simulink library "hapsrav_library"  (R2017a)
settings: Solver=VariableStepAuto  StartTime=0.0  StopTime=10.0  RelTol=1e-3
values from neighbouring files (symbols this model uses):
  absorb_h = 0:100:40000    [EnergySim.m]
  Adisk = pi * v.R_prop^2    [EnergySim.m]
  alpha_h = absorb_h    [EnergySim.m]
  aoa_data = zeros(n_cl, n)    [EnergySim.m]
  cl_bp = linspace(min_cl, max_cl,n_cl)    [EnergySim.m]
  D = [1       -.0065      288.15          0                   101325 ... (first row only)    [EnergySim.m]    (also in msn_params.m = sqrt((from_x - to_x)^2 + (from_y - to_y)^2); solar_vector.m = time.day + ut_time)
  d2r = pi / 180    (= 0.0174532925199)    [EnergySim.m]    (also in example1.m; example2.m; example3.m; example4.m)
  d_init = sqrt(dx*dx + dy*dy)    [EnergySim.m]    (also in msn_init.m)
  dchi0 = atan2(sin(dchi0), cos(dchi0))    [EnergySim.m]    (also in msn_init.m)
  dT = 0.5    [EnergySim.m]
  dT_fixed = 0.5    [EnergySim.m]
  dT_trig = 30    [EnergySim.m]
  earth_rho = 6378137.0    (= 6378137)    [EnergySim.m]
  fp = solarFP(p.orbit_rho, p.min_axis, p.orbit_dir, ic.x_ctr, ic.y_ctr, sun_az_0)    [EnergySim.m]    (also in load_fp.m = gid_tc(msn_idx).fp; solarFP.m = [1	6	2	nul eul 0	0	0	0	1	0)
  fp_coords = [x_entry y_entry]    [msn_params.m]
  fp_courses = [chi_adj nxt_chi dchi]    [msn_params.m]
  g = 9.80665    [EnergySim.m]
  Gsolar = 1367    [EnergySim.m]
  k = k+1    (= 5)    [EnergySim.m]
  K = D(:,2)    [EnergySim.m]
  lat_init = ic.lat_init_deg * obj.d2r    [EnergySim.m]
  M = time.month    [solar_vector.m]
  max_cl = max(cl_data(:))    [EnergySim.m]
  min_cl = min(cl_data(:))    [EnergySim.m]
  ND2 = load(fullfile(pwd,'nd2_data.mat'))    [EnergySim.m]    (also in nd2_data.mat = [0.0999999999999 0.200000000001 0.3 0.4 0.499999999998 0.700)
  next_init = fp(init_wp, 3)    [EnergySim.m]    (also in msn_init.m)
  pE_init = ic.pE_init    [EnergySim.m]
  pN_init = ic.pN_init    [EnergySim.m]
  r2d = 180 / pi    (= 57.2957795131)    [EnergySim.m]    (also in example1.m; example2.m; example3.m; example4.m)
  rho_SL = 1.225    [EnergySim.m]
  S = 110.4    [EnergySim.m]
  thr_lo_lim = 0.0    (= 0)    [EnergySim.m]
  time_init = struct('year', time.year, 'month', time.month,                  'day', time.day, 'hour', time.hour, 'min', time.min,                  'UTC', time.UTC)    [EnergySim.m]
  to_init = fp(init_wp, 1)    [EnergySim.m]    (also in msn_init.m)
  vgnd_init = sqrt(Vg)    [EnergySim.m]
  vtas_init = veas_init * sqrt(rho_sl/rho_alt)    [EnergySim.m]
  w_alt = 2.0 * w_alt    [EnergySim.m]
  w_xtrack = 2.0 * w_xtrack    [EnergySim.m]
undefined symbols (not defined in the file or in its folder): alpha, alpha_bp, alpha_circ, alt0_rate_init, alt_bp, alt_cmd_mode, alt_init, alt_lim_h, alt_lim_l, alt_rt_lim_periodic, cd_data, charge_eff, chi0_rate_init, chi_cmd_mode, chi_inf, chi_init, cl_data, discharge_eff, DiscIntNeverNeededParam, E_batt_max, E_init, Earth, enableFuzzyLogic, entry_init, epsln, epsln_circ, exit_init, f8_azimuth_offset, fig_eight_time, fp0, fp_coords0, fp_courses0, gamma_lim, hold_time, k_c, K_circ, lat_init_deg, lon_init_deg, max_alpha_bp, max_alt_bp, min_alpha_bp, min_alt_bp, min_axis, motor_eff, mppt_eff, num_motors, orb_dir_init, orb_len_init, orbit_dir, orbit_rho, P_acc, panel_eff, panel_vecs, phi_0, phi_lim, phi_lim_alt, phi_lim_alt_max, phi_lim_alt_min, phi_rt_lim, prop_eff_scale ... (+39)
libraries: simulink x59, hapsrav_library x9, fuzblock x3, atmospheric_library x1, aerolibtransform2 x1
(part 2 of 6)

== system hapsrav_library/Cmd - Parametric/Chi Cmd/Subsystem ==
  night_md : Inport
  chi_cmd_in : Inport  Port=2
  sun_az_rad : Inport  Port=3
  Enable : EnablePort  StatesWhenEnabling=reset
  "Azimuth angle not bounded by 0, 2pi" : Subsystem
  Circular Orbit : Subsystem  TreatAsAtomicUnit=on
  Clock : Clock
  Compare To Constant : simulink/Logic and Bit Operations/Compare To Constant  relop===  const=1  OutDataTypeStr=boolean
  Compare To Constant1 : simulink/Logic and Bit Operations/Compare To Constant  relop===  const=2  OutDataTypeStr=boolean
  Compare To Constant2 : simulink/Logic and Bit Operations/Compare To Constant  relop===  const=3  OutDataTypeStr=boolean
  Constant : Constant  Value=chi_cmd_mode
  Constant1 : Constant
  Figure Eight Orbit : Subsystem
  Merge : Merge  Inputs=3
  Racetrack Orbit : Subsystem
  Scope1 : Scope
  Switch : Switch  Criteria=u2 ~= 0
  chi_cmd : Outport
  up_or_down : Outport  Port=2
  wires:
  sun_az_rad/1 -> "Azimuth angle not bounded by 0, 2pi"/1(sun_az_rad), Figure Eight Orbit/2(sun_az_rad), Racetrack Orbit/3(sun_az_rad)
  Constant1/1 -> Switch/1
  Compare To Constant2/1 -> Figure Eight Orbit/Enable
  Constant/1 -> Switch/3
  Figure Eight Orbit/1(chi_cmd) -> Merge/3
  [t] -> Circular Orbit/2(t)
  chi_cmd_in/1 -> Circular Orbit/1(chi_cmd_in), Racetrack Orbit/2(chi_cmd_in), Figure Eight Orbit/3(chi_cmd_in)
  Switch/1 -> Compare To Constant/1, Compare To Constant1/1, Compare To Constant2/1, Scope1/1
  Circular Orbit/1(chi_cmd) -> Merge/1
  Racetrack Orbit/1(chi_cmd) -> Merge/2
  [t] -> Figure Eight Orbit/1(t)
  Compare To Constant1/1 -> Racetrack Orbit/Enable
  Compare To Constant/1 -> Circular Orbit/Enable
  [t] -> Racetrack Orbit/1(t)
  Clock/1 -> [t]
  Merge/1 -> chi_cmd/1
  night_md/1 -> Switch/2
  Racetrack Orbit/2(up_or_down) -> up_or_down/1
  "Azimuth angle not bounded by 0, 2pi"/1(2*pi*i) -> Figure Eight Orbit/4(az_offset)

== system hapsrav_library/Cmd - Parametric/Fuzzy Trajectory Optimiser Alt Cmd/Alt Rate Integrator ==
  alt_rate_cmd : Inport
  alt : Inport  Port=2
  Abs : Abs
  Compare To Constant : simulink/Logic and Bit Operations/Compare To Constant  relop=>  const=50  OutDataTypeStr=boolean
  Delay1 : Delay  DelayLength=1  InitialCondition=alt_init
  Discrete-Time Integrator : DiscreteIntegrator  IntegratorMethod=Integration: Trapezoidal  ExternalReset=rising  InitialConditionSource=external  InitialConditionSetting=State (most efficient)  SampleTime=-1  ICPrevOutput=DiscIntNeverNeededParam  ICPrevScaledInput=DiscIntNeverNeededParam
  Sum : Sum  Inputs=|+-
  alt_cmd : Outport
  wires:
  Delay1/1 -> alt_cmd/1, Discrete-Time Integrator/3, Sum/2
  Discrete-Time Integrator/1 -> Delay1/1
  alt_rate_cmd/1 -> Discrete-Time Integrator/1
  Compare To Constant/1 -> Discrete-Time Integrator/2  "trigger a reset (anti-windup)"
  alt/1 -> Sum/1
  Sum/1 -> Abs/1
  Abs/1 -> Compare To Constant/1

== system hapsrav_library/Cmd - Parametric/Fuzzy Trajectory Optimiser Chi Cmd/Subsystem ==
  chi_rate_cmd_rps : Inport
  chi : Inport  Port=2
  Abs : Abs
  Bus Creator : BusCreator  Inputs=3
  Compare To Constant : simulink/Logic and Bit Operations/Compare To Constant  relop=>  const=1000  OutDataTypeStr=boolean
  Delay1 : Delay  DelayLength=1  InitialCondition=chi_init
  Discrete-Time Integrator : DiscreteIntegrator  IntegratorMethod=Integration: Trapezoidal  ExternalReset=rising  InitialConditionSource=external  InitialConditionSetting=State (most efficient)  SampleTime=-1  ICPrevOutput=DiscIntNeverNeededParam  ICPrevScaledInput=DiscIntNeverNeededParam
  Sum : Sum  Inputs=|+-
  To Workspace1 : ToWorkspace  VariableName=pos_vector  SampleTime=-1
  chi_cmd_rad : Outport
  wires:
  Compare To Constant/1 -> Discrete-Time Integrator/2  "trigger a reset (anti-windup)"
  Sum/1 -> Abs/1
  Discrete-Time Integrator/1 -> Delay1/1
  Abs/1 -> Bus Creator/3, Compare To Constant/1
  Bus Creator/1 -> To Workspace1/1
  chi/1 -> Bus Creator/1, Sum/1
  Delay1/1 -> Discrete-Time Integrator/3, Sum/2, chi_cmd_rad/1, Bus Creator/2
  chi_rate_cmd_rps/1 -> Discrete-Time Integrator/1

== system hapsrav_library/Cmd - Parametric/Wind State/Rel Hdg ==
  wnd_dir : Inport
  psi : Inport  Port=2
  Sum : Sum  Inputs=|+-
  Trigonometric Function6 : Trigonometry
  Trigonometric Function7 : Trigonometry  Operator=cos
  Trigonometric Function8 : Trigonometry  Operator=atan2
  rel_wnd : Outport
  wires:
  Trigonometric Function6/1 -> Trigonometric Function8/1
  wnd_dir/1 -> Sum/1
  Trigonometric Function8/1 -> rel_wnd/1
  Sum/1 -> Trigonometric Function6/1, Trigonometric Function7/1
  Trigonometric Function7/1 -> Trigonometric Function8/2
  psi/1 -> Sum/2

== system hapsrav_library/Winds/Test Winds/Turn winds off at runtime ==
  Action Port : ActionPort
  East : Constant  Value=0.0
  North : Constant  Value=0.0
  Wn : Outport
  We : Outport  Port=2
  wires:
  North/1 -> Wn/1
  East/1 -> We/1

== system hapsrav_library/Winds/Test Winds/Winds ==
  day : Inport
  wmag_level : Inport  Port=2
  wdir_level : Inport  Port=3
  altitude : Inport  Port=4
  Action Port : ActionPort
  Gain : Gain  Gain=pi/180
  Product : Product
  Product1 : Product
  Trigonometric Function : Trigonometry  Operator=sincos
  Wind Direction LUT : Lookup_n-D  NumberOfTableDimensions=3  BreakpointsForDimension1=[1:1:365]  BreakpointsForDimension2=testStation.percs  BreakpointsForDimension3=testStation.alts  Table=testStation.wnd_dir  ExtrapMethod=Clip  UseLastTableValue=on  InternalRulePriority=Speed  RndMeth=Simplest  InputSameDT=on
  Wind Magnitude LUT : Lookup_n-D  NumberOfTableDimensions=3  BreakpointsForDimension1=[1:1:365]  BreakpointsForDimension2=testStation.percs  BreakpointsForDimension3=testStation.alts  Table=testStation.wnd_mag  ExtrapMethod=Clip  UseLastTableValue=on  InternalRulePriority=Speed  RndMeth=Simplest  InputSameDT=on
  Wn : Outport
  We : Outport  Port=2
  wires:
  day/1 -> Wind Direction LUT/1, Wind Magnitude LUT/1
  altitude/1 -> Wind Magnitude LUT/3, Wind Direction LUT/3
  Wind Direction LUT/1 -> Gain/1
  Gain/1 -> Trigonometric Function/1
  Trigonometric Function/2 -> [cos_dir]
  Trigonometric Function/1 -> [sin_dir]
  Wind Magnitude LUT/1 -> [w_mag]
  [w_mag] -> Product/1
  [w_mag] -> Product1/1
  [cos_dir] -> Product/2
  Product/1 -> Wn/1
  [sin_dir] -> Product1/2
  Product1/1 -> We/1
  wmag_level/1 -> Wind Magnitude LUT/2
  wdir_level/1 -> Wind Direction LUT/2

== system hapsrav_library/hapsrav_main/Kinematic 6DOF/Aero ==
  q_bar : Inport
  phi : Inport  Port=2
  gamma : Inport  Port=3
  d1Vtas : Inport  Port=4
  Vtas : Inport  Port=5
  alt : Inport  Port=6
  CL vs AoA : Subsystem
  Constant2 : Constant  Value=S
  Divide1 : Product  Inputs=**
  Thrust : Subsystem
  alpha : Outport
  theta : Outport  Port=2
  thrust : Outport  Port=3
  CL : Outport  Port=4
  CD : Outport  Port=5
  wires:
  d1Vtas/1 -> [d1Vtas]
  Divide1/1 -> [qS]
  gamma/1 -> [gamma]
  q_bar/1 -> [q_bar]
  Constant2/1 -> Divide1/2
  [q_bar] -> Divide1/1
  phi/1 -> [phi]
  Vtas/1 -> [Vtas]
  alt/1 -> [alt]
  [Vtas] -> CL vs AoA/1(Vtas)
  [gamma] -> CL vs AoA/2(gamma)
  CL vs AoA/1(CL) -> [CL]
  CL vs AoA/3(alpha) -> [alpha]
  [qS] -> CL vs AoA/3(qS)
  [alt] -> CL vs AoA/4(alt)
  CL vs AoA/4(theta) -> [theta]
  [d1Vtas] -> Thrust/1(d1Vtas)
  [phi] -> CL vs AoA/5(phi)
  [gamma] -> Thrust/2(gamma)
  [qS] -> Thrust/3(qS)
  [CL] -> Thrust/4(CL)
  Thrust/1(thrust) -> thrust/1
  [CL] -> CL/1
  [alpha] -> alpha/1
  [CD] -> Thrust/5(CD)
  [theta] -> theta/1
  CL vs AoA/2(CD) -> [CD]
  [CD] -> CD/1

== system hapsrav_library/hapsrav_main/Kinematic 6DOF/Airspeed ==
  alt : Inport
  Veas_cmd : Inport  Port=2
  s6dof0 : Inport  Port=3
  Bus Selector : BusSelector  OutputSignals=vtas0
  Constant : Constant  Value=rho_SL
  Delay1 : Delay  DelayLength=1  InitialConditionSource=Input port
      settings: InputPortMap=u0,p4
  Discrete-Time Integrator : DiscreteIntegrator  IntegratorMethod=Integration: Trapezoidal  InitialConditionSource=external  InitialConditionSetting=State (most efficient)  SampleTime=-1  ICPrevOutput=DiscIntNeverNeededParam  ICPrevScaledInput=DiscIntNeverNeededParam
  Divide2 : Product  Inputs=**
  Divide3 : Product  Inputs=**
  Divide4 : Product  Inputs=/*
  Math Function : Math  Operator=square  SaturateOnIntegerOverflow=on
  Mux1 : Mux  Inputs=2
  Saturation : Saturate  UpperLimit=1e3  LowerLimit=-1e3
  Scope : Scope
  Std Atmos : Subsystem
  Sum : Sum  Inputs=|+-
  rho_SL1 : Gain  Gain=0.5
  tau : Gain  Gain=tau_as
  vtas : Outport
  d1vtas : Outport  Port=2
  q_bar : Outport  Port=3
  Veas : Outport  Port=4
  OAT : Outport  Port=5
  wires:
  tau/1 -> Divide3/1
  [vtas0] -> Discrete-Time Integrator/2
  [veas_cmd] -> Mux1/1
  [veas_cmd] -> Sum/1
  Veas_cmd/1 -> [veas_cmd]
  [veas] -> Mux1/2
  Mux1/1 -> Scope/1
  [vtas] -> vtas/1
  [d1vtas] -> d1vtas/1
  Delay1/1 -> Divide4/2
  Divide4/1 -> [veas], Sum/2
  Discrete-Time Integrator/1 -> Delay1/1, [vtas]
  [rho_ratio] -> Divide4/1, Divide3/2
  Bus Selector/1 -> [vtas0]  "<vtas0>"
  s6dof0/1 -> Bus Selector/1
  [vtas0] -> Delay1/2
  Std Atmos/2(OAT) -> OAT/1
  [veas] -> Veas/1
  Std Atmos/1(rho_ratio) -> [rho_ratio]
  Constant/1 -> Divide2/2
  alt/1 -> Std Atmos/1(alt)
  rho_SL1/1 -> q_bar/1
  Divide2/1 -> rho_SL1/1
  Math Function/1 -> Divide2/1
  [veas] -> Math Function/1
  Sum/1 -> tau/1
  Divide3/1 -> Saturation/1
  Saturation/1 -> [d1vtas], Discrete-Time Integrator/1

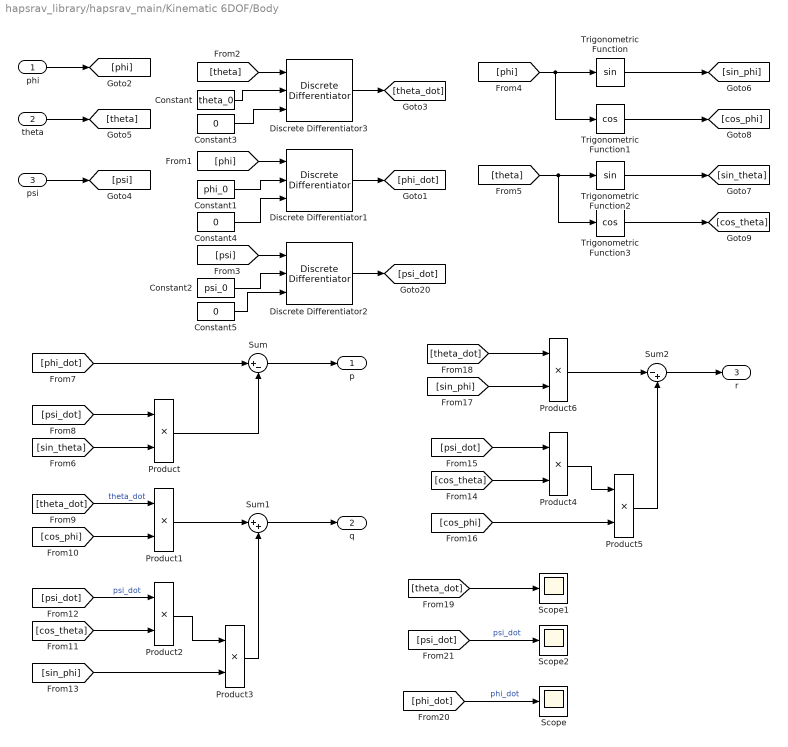
== system hapsrav_library/hapsrav_main/Kinematic 6DOF/Body ==
  phi : Inport
  theta : Inport  Port=2
  psi : Inport  Port=3
  Constant : Constant  Value=theta_0
  Constant1 : Constant  Value=phi_0
  Constant2 : Constant  Value=psi_0
  Constant3 : Constant  Value=0
  Constant4 : Constant  Value=0
  Constant5 : Constant  Value=0
  Discrete Differentiator1 : hapsrav_library/Discrete Differentiator
  Discrete Differentiator2 : hapsrav_library/Discrete Differentiator
  Discrete Differentiator3 : hapsrav_library/Discrete Differentiator
  Product{,1..6} (7 alike) : Product
  Scope : Scope
  Scope1 : Scope
  Scope2 : Scope
  Sum : Sum  Inputs=|+-
  Sum1 : Sum  Inputs=|++
  Sum2 : Sum  Inputs=|-+
  Trigonometric Function : Trigonometry
  Trigonometric Function1 : Trigonometry  Operator=cos
  Trigonometric Function2 : Trigonometry
  Trigonometric Function3 : Trigonometry  Operator=cos
  p : Outport
  q : Outport  Port=2
  r : Outport  Port=3
  wires:
  [theta_dot] -> Scope1/1
  Constant5/1 -> Discrete Differentiator2/3
  Constant4/1 -> Discrete Differentiator1/3
  Constant3/1 -> Discrete Differentiator3/3
  [psi_dot] -> Scope2/1  "psi_dot"
  [phi_dot] -> Scope/1  "phi_dot"
  Constant/1 -> Discrete Differentiator3/2
  psi/1 -> [psi]
  theta/1 -> [theta]
  phi/1 -> [phi]
  [phi] -> Trigonometric Function1/1, Trigonometric Function/1
  [theta] -> Trigonometric Function3/1, Trigonometric Function2/1
  Trigonometric Function3/1 -> [cos_theta]
  Trigonometric Function2/1 -> [sin_theta]
  Trigonometric Function1/1 -> [cos_phi]
  Trigonometric Function/1 -> [sin_phi]
  [sin_theta] -> Product/2
  [psi_dot] -> Product/1
  [phi_dot] -> Sum/1
  Product/1 -> Sum/2
  Sum/1 -> p/1
  [theta_dot] -> Product1/1  "theta_dot"
  [cos_phi] -> Product1/2
  [cos_theta] -> Product2/2
  [psi_dot] -> Product2/1  "psi_dot"
  Product2/1 -> Product3/1
  [sin_phi] -> Product3/2
  Product1/1 -> Sum1/1
  Product3/1 -> Sum1/2
  Sum1/1 -> q/1
  [cos_theta] -> Product4/2
  [psi_dot] -> Product4/1
  Product4/1 -> Product5/1
  [cos_phi] -> Product5/2
  Product5/1 -> Sum2/2
  [theta_dot] -> Product6/1
  [sin_phi] -> Product6/2
  Product6/1 -> Sum2/1
  Sum2/1 -> r/1
  Discrete Differentiator3/1 -> [theta_dot]
  [theta] -> Discrete Differentiator3/1
  [phi] -> Discrete Differentiator1/1
  Constant1/1 -> Discrete Differentiator1/2
  Discrete Differentiator1/1 -> [phi_dot]
  Constant2/1 -> Discrete Differentiator2/2
  [psi] -> Discrete Differentiator2/1
  Discrete Differentiator2/1 -> [psi_dot]

== system hapsrav_library/hapsrav_main/Kinematic 6DOF/EAS Cmd Filter ==
  eas cmd : Inport
  s6dof0 : Inport  Port=2
  1/tau : Gain  Gain=0.1
  Bus Selector : BusSelector  OutputSignals=veas0
  Delay1 : Delay  DelayLength=1  InitialConditionSource=Input port
      settings: InputPortMap=u0,p4
  Discrete-Time Integrator : DiscreteIntegrator  IntegratorMethod=Integration: Trapezoidal  InitialConditionSource=external  InitialConditionSetting=State (most efficient)  SampleTime=-1  ICPrevOutput=DiscIntNeverNeededParam  ICPrevScaledInput=DiscIntNeverNeededParam
  Saturation : Saturate  UpperLimit=veas_rt_lim  LowerLimit=-veas_rt_lim
  Sum : Sum  Inputs=|+-
  filt eas cmd : Outport
  wires:
  Saturation/1 -> Discrete-Time Integrator/1
  1/tau/1 -> Saturation/1
  Sum/1 -> 1/tau/1
  Discrete-Time Integrator/1 -> filt eas cmd/1, Delay1/1
  eas cmd/1 -> Sum/1
  Delay1/1 -> Sum/2
  [eas_init] -> Discrete-Time Integrator/2
  [eas_init] -> Delay1/2
  Bus Selector/1 -> [eas_init]  "<veas0>"
  s6dof0/1 -> Bus Selector/1

== system hapsrav_library/hapsrav_main/Kinematic 6DOF/Idle Pwr ==
  thrust : Inport
  hdot : Inport  Port=2
  vdot : Inport  Port=3
  Constant1 : Constant  Value=THRUST_REVERSAL
  Constant2 : Constant  Value=thrust0
  Data Type Conversion : DataTypeConversion  OutDataTypeStr=double
  Data Type Conversion1 : DataTypeConversion  OutDataTypeStr=double
  Decel Detection : Stateflow chart  TreatAsAtomicUnit=on
  Delay1 : Delay  DelayLength=1  InitialConditionSource=Input port
      settings: InputPortMap=u0,p4
  Descent Detection : Stateflow chart  TreatAsAtomicUnit=on
  Logical Operator : Logic  Operator=NOT  AllPortsSameDT=off  OutDataTypeStr=boolean
  Logical Operator1 : Logic  AllPortsSameDT=off  OutDataTypeStr=boolean
  Logical Operator2 : Logic  AllPortsSameDT=off  OutDataTypeStr=boolean
  Scope : Scope
  Scope1 : Scope  NumInputPorts=2
  Terminator : Terminator
  Terminator1 : Terminator
  idleDesc : Outport
  wires:
  Data Type Conversion1/1 -> idleDesc/1
  Data Type Conversion/1 -> Terminator1/1
  Logical Operator1/1 -> Data Type Conversion/1
  [idle_descent] -> Logical Operator2/2
  Logical Operator2/1 -> Data Type Conversion1/1
  [idle_decel] -> Logical Operator1/1
  Logical Operator/1 -> Logical Operator2/1, Logical Operator1/2
  [idle_decel] -> Scope1/1
  Descent Detection/2(idleDesc) -> [idle_descent]
  Constant1/1 -> Logical Operator/1
  [thrust] -> Scope1/2
  Decel Detection/1(spd_flag) -> Scope/1
  Decel Detection/2(idleDecel) -> [idle_decel]
  [thrust] -> Decel Detection/2(thrust)
  [vdot] -> Decel Detection/1(vdot)
  Descent Detection/1(alt_flag) -> Terminator/1
  [hdot] -> Descent Detection/1(hdot)
  [thrust] -> Descent Detection/2(thrust)
  Delay1/1 -> [thrust]
  Constant2/1 -> Delay1/2
  thrust/1 -> Delay1/1
  hdot/1 -> [hdot]
  vdot/1 -> [vdot]

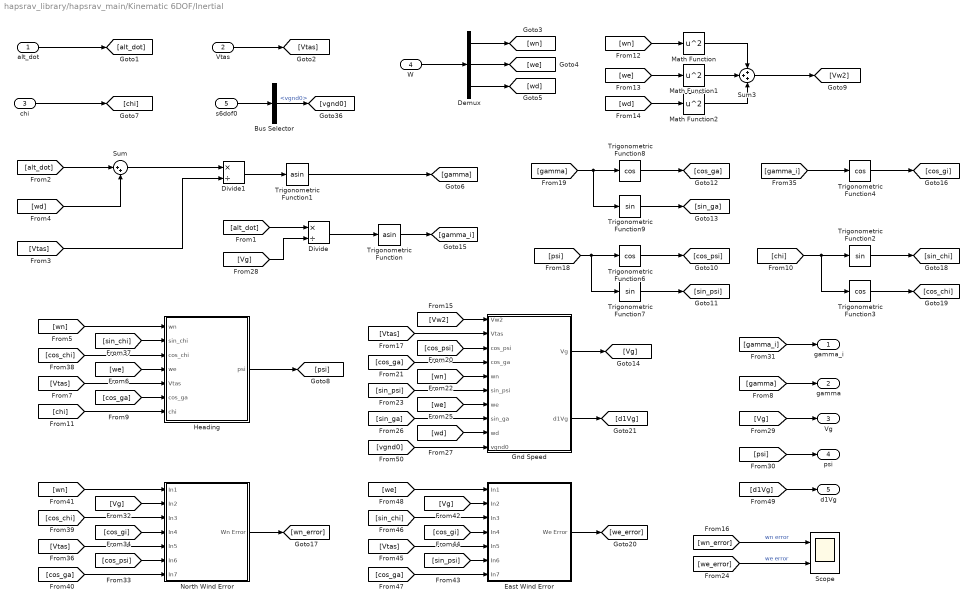
== system hapsrav_library/hapsrav_main/Kinematic 6DOF/Inertial ==
  alt_dot : Inport
  Vtas : Inport  Port=2
  chi : Inport  Port=3
  W : Inport  Port=4
  s6dof0 : Inport  Port=5
  Bus Selector : BusSelector  OutputSignals=vgnd0
  Demux : Demux  Outputs=3
  Divide : Product  Inputs=*/
  Divide1 : Product  Inputs=*/
  East Wind Error : Subsystem
  Gnd Speed : Subsystem
  Heading : Subsystem
  Math Function : Math  Operator=square  SaturateOnIntegerOverflow=on
  Math Function1 : Math  Operator=square  SaturateOnIntegerOverflow=on
  Math Function2 : Math  Operator=square  SaturateOnIntegerOverflow=on
  North Wind Error : Subsystem
  Scope : Scope  NumInputPorts=2
  Sum : Sum  Inputs=|++
  Sum3 : Sum  Inputs=+++
  Trigonometric Function : Trigonometry  Operator=asin
  Trigonometric Function1 : Trigonometry  Operator=asin
  Trigonometric Function2 : Trigonometry
  Trigonometric Function{3..4,6,8} (4 alike) : Trigonometry  Operator=cos
  Trigonometric Function7 : Trigonometry
  Trigonometric Function9 : Trigonometry
  gamma_i : Outport
  gamma : Outport  Port=2
  Vg : Outport  Port=3
  psi : Outport  Port=4
  d1Vg : Outport  Port=5
  wires:
  [Vg] -> Divide/2
  Divide/1 -> Trigonometric Function/1
  alt_dot/1 -> [alt_dot]
  [alt_dot] -> Divide/1
  [alt_dot] -> Sum/1
  [wd] -> Sum/2
  Sum/1 -> Divide1/1
  Vtas/1 -> [Vtas]
  [Vtas] -> Divide1/2
  Divide1/1 -> Trigonometric Function1/1
  Trigonometric Function1/1 -> [gamma]
  W/1 -> Demux/1
  Demux/1 -> [wn]
  Demux/2 -> [we]
  Demux/3 -> [wd]
  [gamma] -> gamma/1
  chi/1 -> [chi]
  [chi] -> Trigonometric Function3/1, Trigonometric Function2/1
  [wn] -> Math Function/1
  [we] -> Math Function1/1
  [wd] -> Math Function2/1
  Math Function/1 -> Sum3/1
  Math Function1/1 -> Sum3/2
  Math Function2/1 -> Sum3/3
  Sum3/1 -> [Vw2]
  [psi] -> Trigonometric Function7/1, Trigonometric Function6/1
  Trigonometric Function6/1 -> [cos_psi]
  Trigonometric Function7/1 -> [sin_psi]
  Trigonometric Function8/1 -> [cos_ga]
  Trigonometric Function9/1 -> [sin_ga]
  [gamma] -> Trigonometric Function9/1, Trigonometric Function8/1
  [Vg] -> Vg/1
  [psi] -> psi/1
  Trigonometric Function/1 -> [gamma_i]
  [gamma_i] -> gamma_i/1
  Trigonometric Function4/1 -> [cos_gi]
  [gamma_i] -> Trigonometric Function4/1
  Trigonometric Function2/1 -> [sin_chi]
  Trigonometric Function3/1 -> [cos_chi]
  [wn] -> Heading/1(wn)
  [sin_chi] -> Heading/2(sin_chi)
  [cos_chi] -> Heading/3(cos_chi)
  [we] -> Heading/4(we)
  [Vtas] -> Heading/5(Vtas)
  [cos_ga] -> Heading/6(cos_ga)
  [chi] -> Heading/7(chi)
  Heading/1(psi) -> [psi]
  [Vw2] -> Gnd Speed/1(Vw2)
  [Vtas] -> Gnd Speed/2(Vtas)
  [cos_psi] -> Gnd Speed/3(cos_psi)
  [cos_ga] -> Gnd Speed/4(cos_ga)
  [wn] -> Gnd Speed/5(wn)
  [sin_psi] -> Gnd Speed/6(sin_psi)
  [we] -> Gnd Speed/7(we)
  [sin_ga] -> Gnd Speed/8(sin_ga)
  [wd] -> Gnd Speed/9(wd)
  Gnd Speed/1(Vg) -> [Vg]
  [wn] -> North Wind Error/1(In1)
  [Vg] -> North Wind Error/2(In2)
  [cos_chi] -> North Wind Error/3(In3)
  [cos_gi] -> North Wind Error/4(In4)
  [Vtas] -> North Wind Error/5(In5)
  [cos_psi] -> North Wind Error/6(In6)
  [cos_ga] -> North Wind Error/7(In7)
  [sin_psi] -> East Wind Error/6(In6)
  [cos_ga] -> East Wind Error/7(In7)
  [Vtas] -> East Wind Error/5(In5)
  [cos_gi] -> East Wind Error/4(In4)
  [sin_chi] -> East Wind Error/3(In3)
  [Vg] -> East Wind Error/2(In2)
  [we] -> East Wind Error/1(In1)
  North Wind Error/1(Wn Error) -> [wn_error]
  East Wind Error/1(We Error) -> [we_error]
  [wn_error] -> Scope/1  "wn error"
  [we_error] -> Scope/2  "we error"
  Gnd Speed/2(d1Vg) -> [d1Vg]
  [d1Vg] -> d1Vg/1
  [vgnd0] -> Gnd Speed/10(vgnd0)
  Bus Selector/1 -> [vgnd0]  "<vgnd0>"
  s6dof0/1 -> Bus Selector/1

== system hapsrav_library/hapsrav_main/Kinematic 6DOF/Initial Conditions ==
  Bus Creator : BusCreator  Inputs='alt0','veas0','phi0','theta0','chi0','vgnd0','altRt0','vtas0'
  Constant : Constant  Value=pE_init
  Constant1 : Constant  Value=alt_init
  Constant10 : Constant  Value=theta_0
  Constant2 : Constant  Value=veas_init
  Constant3 : Constant  Value=chi_init
  Constant4 : Constant  Value=vgnd_init
  Constant5 : Constant  Value=vtas_init
  Constant7 : Constant  Value=alt0_rate_init
  Constant8 : Constant  Value=pN_init
  Constant9 : Constant  Value=phi_0
  Mux : Mux  Inputs=2
  s6dof0 : Outport
  posn0 : Outport  Port=2
  wires:
  Constant5/1 -> Bus Creator/8  "vtas0"
  Constant8/1 -> Mux/2  "pN_0"
  Constant/1 -> Mux/1  "pE_0"
  Bus Creator/1 -> s6dof0/1
  Constant1/1 -> Bus Creator/1  "alt0"
  Constant2/1 -> Bus Creator/2  "veas0"
  Constant9/1 -> Bus Creator/3  "phi0"
  Constant10/1 -> Bus Creator/4  "theta0"
  Constant3/1 -> Bus Creator/5  "chi0"
  Constant4/1 -> Bus Creator/6  "vgnd0"
  Constant7/1 -> Bus Creator/7  "altRt0"
  Mux/1 -> posn0/1

== system hapsrav_library/hapsrav_main/Kinematic 6DOF/Navigation ==
  Va : Inport
  psi : Inport  Port=2
  W : Inport  Port=3
  alt : Inport  Port=4
  posn0 : Inport  Port=5
  Demux : Demux  Outputs=3
  Demux1 : Demux  Outputs=2
  Flat Earth to LLA : Subsystem  Commented=on
  Flat Earth to LLA Aero BLockset : Subsystem
  NED Posn : Subsystem
  Terminator : Terminator
  Terminator3 : Terminator
  Terminator4 : Terminator
  pN : Outport
  pE : Outport  Port=2
  lat_deg : Outport  Port=3
  lon_deg : Outport  Port=4
  wires:
  Va/1 -> [Va]
  psi/1 -> [psi]
  W/1 -> Demux/1
  Demux/1 -> [wn]
  Demux/2 -> [we]
  Demux/3 -> Terminator/1
  [Va] -> NED Posn/1(Va)
  [psi] -> NED Posn/2(psi)
  [we] -> NED Posn/3(we)
  [wn] -> NED Posn/4(wn)
  NED Posn/2(pE_dot) -> Terminator3/1
  NED Posn/4(pN_dot) -> Terminator4/1
  alt/1 -> [alt]
  Demux1/1 -> NED Posn/5(pE0)
  Demux1/2 -> NED Posn/6(pN0)
  NED Posn/1(pE) -> [pE]
  NED Posn/3(pN) -> [pN]
  [pE] -> pE/1
  [pN] -> pN/1
  Flat Earth to LLA Aero BLockset/1(lat_deg) -> lat_deg/1
  [alt] -> Flat Earth to LLA Aero BLockset/1(alt)
  [pN] -> Flat Earth to LLA Aero BLockset/2(pN)
  [pE] -> Flat Earth to LLA Aero BLockset/3(pE)
  Flat Earth to LLA Aero BLockset/2(lon_deg) -> lon_deg/1
  posn0/1 -> Demux1/1

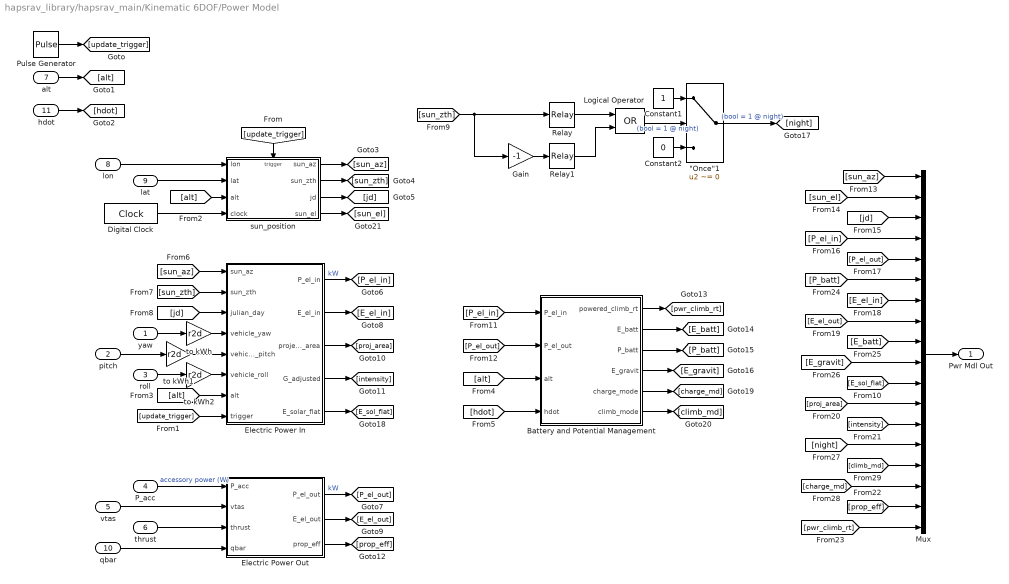
== system hapsrav_library/hapsrav_main/Kinematic 6DOF/Power Model ==
  yaw : Inport
  pitch : Inport  Port=2
  roll : Inport  Port=3
  P_acc : Inport  Port=4
  vtas : Inport  Port=5
  thrust : Inport  Port=6
  alt : Inport  Port=7
  lon : Inport  Port=8
  lat : Inport  Port=9
  qbar : Inport  Port=10
  hdot : Inport  Port=11
  "\"Once\"1" : Switch  Criteria=u2 ~= 0
  Battery and Potential Management : Subsystem
  Constant1 : Constant
  Constant2 : Constant  Value=0
  Digital Clock : DigitalClock  SampleTime=dT_fixed
  Electric Power In : Subsystem
  Electric Power Out : Subsystem
  Gain : Gain  Gain=-1
  Logical Operator : Logic  Operator=OR  AllPortsSameDT=off  OutDataTypeStr=boolean
  Mux : Mux  Inputs=18
  Pulse Generator : DiscretePulseGenerator  Period=dT_trig*2/dT_fixed  PulseWidth=dT_trig/dT_fixed  PhaseDelay=1  SampleTime=dT_fixed
  Relay : Relay  OnSwitchValue=90  OffSwitchValue=89.5
  Relay1 : Relay  OnSwitchValue=90  OffSwitchValue=89.5
  sun_position : Subsystem  TreatAsAtomicUnit=on
  to kWh : Gain  Gain=r2d
  to kWh1 : Gain  Gain=r2d
  to kWh2 : Gain  Gain=r2d
  Pwr Mdl Out : Outport
  wires:
  roll/1 -> to kWh2/1
  yaw/1 -> to kWh/1
  P_acc/1 -> Electric Power Out/1(P_acc)  "accessory power (W)"
  Battery and Potential Management/1(powered_climb_rt) -> [pwr_climb_rt]
  vtas/1 -> Electric Power Out/2(vtas)
  pitch/1 -> to kWh1/1
  lon/1 -> sun_position/1(lon)
  lat/1 -> sun_position/2(lat)
  to kWh/1 -> Electric Power In/4(vehicle_yaw)
  to kWh1/1 -> Electric Power In/5(vehicle_pitch)
  to kWh2/1 -> Electric Power In/6(vehicle_roll)
  qbar/1 -> Electric Power Out/4(qbar)
  Digital Clock/1 -> sun_position/4(clock)
  Pulse Generator/1 -> [update_trigger]
  [update_trigger] -> sun_position/Trigger
  [update_trigger] -> Electric Power In/8(trigger)
  alt/1 -> [alt]
  [alt] -> sun_position/3(alt)
  [alt] -> Electric Power In/7(alt)
  [alt] -> Battery and Potential Management/3(alt)
  "\"Once\"1"/1 -> [night]  "(bool = 1 @ night)"
  Relay1/1 -> Logical Operator/2
  Relay/1 -> Logical Operator/1
  Gain/1 -> Relay1/1
  Constant1/1 -> "\"Once\"1"/1
  Constant2/1 -> "\"Once\"1"/3
  Logical Operator/1 -> "\"Once\"1"/2  "(bool = 1 @ night)"
  hdot/1 -> [hdot]
  [hdot] -> Battery and Potential Management/4(hdot)
  thrust/1 -> Electric Power Out/3(thrust)
  sun_position/1(sun_az) -> [sun_az]
  sun_position/3(jd) -> [jd]
  sun_position/2(sun_zth) -> [sun_zth]
  [sun_az] -> Electric Power In/1(sun_az)
  [sun_zth] -> Electric Power In/2(sun_zth)
  [jd] -> Electric Power In/3(julian_day)
  [sun_zth] -> Gain/1, Relay/1
  Electric Power In/1(P_el_in) -> [P_el_in]  "kW"
  Electric Power Out/1(P_el_out) -> [P_el_out]  "kW"
  [P_el_in] -> Battery and Potential Management/1(P_el_in)
  [P_el_out] -> Battery and Potential Management/2(P_el_out)
  Electric Power In/2(E_el_in) -> [E_el_in]
  Electric Power Out/2(E_el_out) -> [E_el_out]
  Electric Power In/3(projected_area) -> [proj_area]
  Electric Power In/4(G_adjusted) -> [intensity]
  Electric Power Out/3(prop_eff) -> [prop_eff]
  Battery and Potential Management/2(E_batt) -> [E_batt]
  Battery and Potential Management/3(P_batt) -> [P_batt]
  Battery and Potential Management/4(E_gravit) -> [E_gravit]
  Mux/1 -> Pwr Mdl Out/1
  Electric Power In/5(E_solar_flat) -> [E_sol_flat]
  Battery and Potential Management/6(climb_mode) -> [climb_md]
  Battery and Potential Management/5(charge_mode) -> [charge_md]
  sun_position/4(sun_el) -> [sun_el]
  [sun_az] -> Mux/1
  [sun_el] -> Mux/2
  [jd] -> Mux/3
  [P_el_in] -> Mux/4
  [P_el_out] -> Mux/5
  [P_batt] -> Mux/6
  [E_el_in] -> Mux/7
  [E_el_out] -> Mux/8
  [E_batt] -> Mux/9
  [E_gravit] -> Mux/10
  [E_sol_flat] -> Mux/11
  [proj_area] -> Mux/12
  [intensity] -> Mux/13
  [night] -> Mux/14
  [climb_md] -> Mux/15
  [charge_md] -> Mux/16
  [prop_eff] -> Mux/17
  [pwr_climb_rt] -> Mux/18

== system hapsrav_library/hapsrav_main/Kinematic 6DOF/Selectable Modes ==
  mode : Inport
  vl_cmds : Inport  Port=2
  Vg : Inport  Port=3
  d1Vg : Inport  Port=4
  s6dof0 : Inport  Port=5
  idleDesc : Inport  Port=6
  Constant2 : Constant  Value=gamma_lim
  Divide : Product  Inputs=**
  Gain : Gain  Gain=-1
  Logical Operator : Logic  Operator=NOT  AllPortsSameDT=off  OutDataTypeStr=boolean
  Merge : Merge  InitialOutput=alt_init
  Merge1 : Merge  InitialOutput=alt0_rate_init
  Merge2 : Merge  InitialOutput=phi_0
  Merge3 : Merge  InitialOutput=chi_init
  Trajectory_Optimization : Subsystem  TreatAsAtomicUnit=on
  Trigonometric Function : Trigonometry
  Waypoint_Navigation : Subsystem  TreatAsAtomicUnit=on
  alt : Outport
  d1alt : Outport  Port=2
  phi : Outport  Port=3
  chi : Outport  Port=4
  wires:
  [idleDesc] -> Waypoint_Navigation/7(idleDesc)
  [max_desc_rt] -> Waypoint_Navigation/6(max_desc_rt)
  [max_desc_rt] -> Trajectory_Optimization/5(max_desc_rt)
  [Vg] -> Divide/2
  Trigonometric Function/1 -> Divide/1
  Divide/1 -> [max_desc_rt], Gain/1
  Constant2/1 -> Trigonometric Function/1
  idleDesc/1 -> [idleDesc]
  [idleDesc] -> Trajectory_Optimization/6(idleDesc)
  mode/1 -> Logical Operator/1, Waypoint_Navigation/Enable
  Logical Operator/1 -> Trajectory_Optimization/Enable
  Trajectory_Optimization/4(chi) -> [b_chi]
  Trajectory_Optimization/1(alt) -> [b_alt]
  Trajectory_Optimization/2(d1alt) -> [b_d1alt]
  Trajectory_Optimization/3(phi) -> [b_phi]
  Waypoint_Navigation/1(alt) -> [a_alt]
  Waypoint_Navigation/2(d1alt) -> [a_d1alt]
  Waypoint_Navigation/3(phi) -> [a_phi]
  Waypoint_Navigation/4(chi) -> [a_chi]
  Merge/1 -> alt/1
  Merge1/1 -> d1alt/1
  Merge2/1 -> phi/1
  Merge3/1 -> chi/1
  [a_alt] -> Merge/1
  [b_alt] -> Merge/2
  [b_d1alt] -> Merge1/2
  [a_d1alt] -> Merge1/1
  [a_phi] -> Merge2/1
  [b_phi] -> Merge2/2
  [b_chi] -> Merge3/2
  [a_chi] -> Merge3/1
  vl_cmds/1 -> [vl_cmds]
  Vg/1 -> [Vg]
  d1Vg/1 -> [d1Vg]
  [vl_cmds] -> Waypoint_Navigation/1(vert_lat_cmds)
  [Vg] -> Waypoint_Navigation/2(Vg)
  [d1Vg] -> Waypoint_Navigation/3(d1Vg)
  [max_clmb_rt] -> Trajectory_Optimization/4(max_clmb_rt)
  [Vg] -> Trajectory_Optimization/2(Vg)
  [vl_cmds] -> Trajectory_Optimization/1(vert_lat_cmds)
  s6dof0/1 -> [ICs]
  [ICs] -> Trajectory_Optimization/3(s6dof0)
  [ICs] -> Waypoint_Navigation/4(s6dof0)
  [max_clmb_rt] -> Waypoint_Navigation/5(max_clmb_rt)
  Gain/1 -> [max_clmb_rt]

== system hapsrav_library/hapsrav_main/Outputs/Negative Gnd Speed ==
  psi : Inport
  gamma : Inport  Port=2
  Vtas : Inport  Port=3
  Vg : Inport  Port=4
  Abs : Abs
  Compare To Constant : simulink/Logic and Bit Operations/Compare To Constant  relop=>  const=pi/2  OutDataTypeStr=boolean
  Compare To Constant1 : simulink/Logic and Bit Operations/Compare To Constant  relop=<=  const=Wmag  OutDataTypeStr=boolean
  Constant : Constant  Value=-1
  Constant1 : Constant  Value=Wmag
  Constant2 : Constant  Value=Wn
  Constant3 : Constant
  Constant4 : Constant  Value=We
  Constant5 : Constant  Value=Wd
  Divide : Product  Inputs=*/
  Divide1 : Product  Inputs=**
  Dot Product : DotProduct  InputSameDT=on  OutDataTypeStr=Inherit: Inherit via internal rule
  Gain : Gain  Gain=-1
  Logical Operator1 : Logic  AllPortsSameDT=off  OutDataTypeStr=boolean
  Mux : Mux  Inputs=3
  Mux1 : Mux  Inputs=3
  Product{,1..3} (4 alike) : Product
  Reshape : Reshape  OutputDimensionality=Row vector (2-D)
  Scope : Scope
  Switch : Switch  Criteria=u2 > Threshold
  Trigonometric Function : Trigonometry  Operator=sincos
  Trigonometric Function4 : Trigonometry  Operator=acos
  Trigonometric Function5 : Trigonometry  Operator=sincos
  Vg_out : Outport
  wires:
  psi/1 -> Trigonometric Function/1
  gamma/1 -> Trigonometric Function5/1
  Trigonometric Function5/1 -> Gain/1
  Gain/1 -> Mux/3
  Mux/1 -> Product2/2
  Product2/1 -> Dot Product/1
  Dot Product/1 -> Divide/1
  Vtas/1 -> [Vtas]
  [Vtas] -> Product2/1
  [Vtas] -> Divide1/1
  Divide1/1 -> Divide/2
  Constant1/1 -> Divide1/2
  Divide/1 -> Trigonometric Function4/1
  Trigonometric Function5/2 -> Product/2, Product1/1
  Trigonometric Function4/1 -> Abs/1
  Abs/1 -> Compare To Constant/1
  [Vtas] -> Compare To Constant1/1
  Compare To Constant1/1 -> Scope/1, Logical Operator1/2
  Compare To Constant/1 -> Logical Operator1/1
  Logical Operator1/1 -> Switch/2
  Constant/1 -> Switch/1
  Constant3/1 -> Switch/3
  Switch/1 -> Product3/2
  Vg/1 -> Product3/1
  Product3/1 -> Vg_out/1
  Trigonometric Function/2 -> Product/1
  Trigonometric Function/1 -> Product1/2
  Product1/1 -> Mux/2
  Product/1 -> Mux/1
  Mux1/1 -> Reshape/1
  Constant2/1 -> Mux1/1
  Constant4/1 -> Mux1/2
  Constant5/1 -> Mux1/3
  Reshape/1 -> Dot Product/2

== system hapsrav_library/Cmd - Parametric/Chi Cmd/Flight Plan/D2N ==
  leg_state : Inport
  av_state : Inport  Port=2
  Bus Selector : BusSelector  OutputSignals=av_posn
  Bus Selector1 : BusSelector  OutputSignals=leg_coords.to_x,leg_coords.to_y
  Demux1 : Demux
  Display1 : Display
  Distance : Subsystem  TreatAsAtomicUnit=on
  Memory5 : Memory  X0=d_init
  Terminator2 : Terminator
  Terminator3 : Terminator
  av_d2n : Outport
  wires:
  [to_y] -> Distance/3(to_y)
  [av_y] -> Distance/4(from_y)
  [av_x] -> Distance/2(from_x)
  [to_x] -> Distance/1(to_x)
  Bus Selector1/1 -> [to_x]  "<to_x>"
  Bus Selector1/2 -> [to_y]  "<to_y>"
  leg_state/1 -> Bus Selector1/1
  Memory5/1 -> av_d2n/1
  Demux1/4 -> Terminator3/1
  Demux1/3 -> Terminator2/1
  [av_d2n] -> Memory5/1
  Bus Selector/1 -> Demux1/1  "<av_posn>"
  av_state/1 -> Bus Selector/1
  Demux1/1 -> [av_x]
  Demux1/2 -> [av_y]
  Distance/1(Dist) -> Display1/1, [av_d2n]

== system hapsrav_library/Cmd - Parametric/Chi Cmd/Flight Plan/Mission Command ==
  orbit_state : Inport
  leg_state : Inport  Port=2
  av_state : Inport  Port=3
  nav_mode : Inport  Port=4
  Compare To Zero : simulink/Logic and Bit Operations/Compare To Zero  relop===  OutDataTypeStr=boolean
  Compare To Zero1 : simulink/Logic and Bit Operations/Compare To Zero  relop=>  OutDataTypeStr=boolean
  Entry Mode : Subsystem
  Merge{,1..3} (4 alike) : Merge
  Not Entry Mode : Subsystem
  Terminator : Terminator
  chi_cmd : Outport
  chi_d : Outport  Port=2
  sweep : Outport  Port=3
  wires:
  [sweep_1] -> Merge3/2
  [sweep_0] -> Merge3/1
  Merge3/1 -> sweep/1
  Not Entry Mode/4(sweep) -> [sweep_1]
  Entry Mode/4(sweep) -> [sweep_0]
  [orbit_state] -> Not Entry Mode/1(orbit_state)
  orbit_state/1 -> [orbit_state]
  [nav_mode] -> Not Entry Mode/4(nav_mode)
  [av_state] -> Not Entry Mode/3(av_state)
  [xtrack_1] -> Merge2/2
  [xtrack_0] -> Merge2/1
  [chi_d_1] -> Merge1/2
  [chi_cmd_1] -> Merge/2
  Not Entry Mode/3(xtrack) -> [xtrack_1]
  Not Entry Mode/2(chi_d) -> [chi_d_1]
  Not Entry Mode/1(chi_cmd) -> [chi_cmd_1]
  [chi_d_0] -> Merge1/1
  [chi_cmd_0] -> Merge/1
  Entry Mode/3(xtrack) -> [xtrack_0]
  Entry Mode/2(chi_d) -> [chi_d_0]
  Entry Mode/1(chi_cmd) -> [chi_cmd_0]
  Merge2/1 -> Terminator/1
  Merge1/1 -> chi_d/1
  Merge/1 -> chi_cmd/1
  [av_state] -> Entry Mode/2(av_state)
  [leg_state] -> Entry Mode/1(leg_state)
  Compare To Zero/1 -> Entry Mode/Enable
  [nav_mode] -> Compare To Zero1/1
  [nav_mode] -> Compare To Zero/1
  Compare To Zero1/1 -> Not Entry Mode/Enable
  nav_mode/1 -> [nav_mode]
  [leg_state] -> Not Entry Mode/2(leg_state)
  leg_state/1 -> [leg_state]
  av_state/1 -> [av_state]

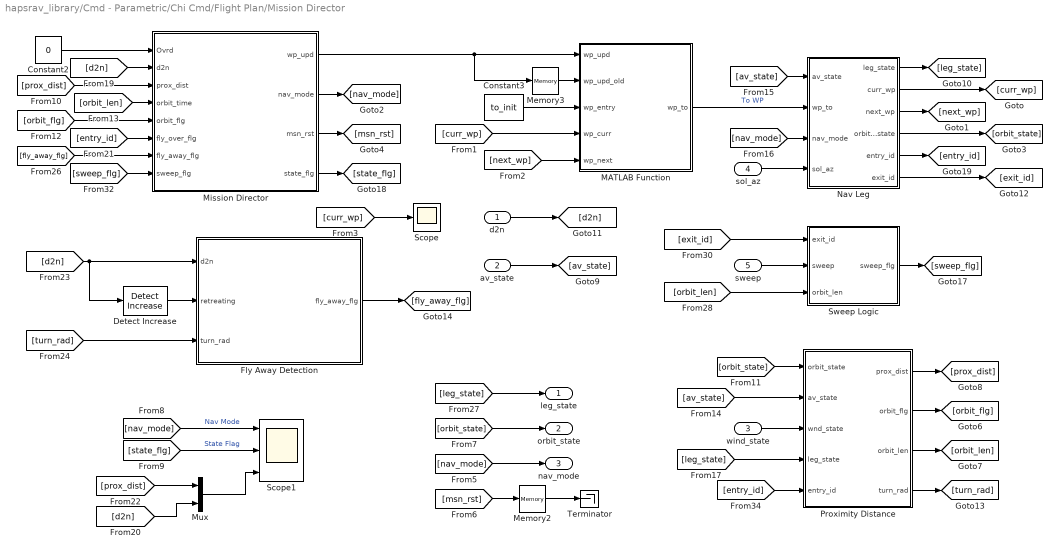
== system hapsrav_library/Cmd - Parametric/Chi Cmd/Flight Plan/Mission Director ==
  d2n : Inport
  av_state : Inport  Port=2
  wind_state : Inport  Port=3
  sol_az : Inport  Port=4
  sweep : Inport  Port=5
  Constant2 : Constant  Value=0
  Constant3 : Constant  Value=to_init
  Detect Increase : simulink/Logic and Bit Operations/Detect Increase  vinit=0.0  OutDataTypeStr=boolean
  Fly Away Detection : Stateflow chart  TreatAsAtomicUnit=on
  MATLAB Function : MATLAB Function  TreatAsAtomicUnit=on
  Memory2 : Memory  X0=1
  Memory3 : Memory  X0=-1
  Mission Director : Stateflow chart  TreatAsAtomicUnit=on
  Mux : Mux  Inputs=2
  Nav Leg : Subsystem
  Proximity Distance : Subsystem
  Scope : Scope
  Scope1 : Scope  NumInputPorts=3
  Sweep Logic : Subsystem
  Terminator : Terminator
  leg_state : Outport
  orbit_state : Outport  Port=2
  nav_mode : Outport  Port=3
  wires:
  Memory2/1 -> Terminator/1
  sol_az/1 -> Nav Leg/4(sol_az)
  [curr_wp] -> Scope/1
  Fly Away Detection/1(fly_away_flg) -> [fly_away_flg]
  Sweep Logic/1(sweep_flg) -> [sweep_flg]
  [orbit_len] -> Sweep Logic/3(orbit_len)
  sweep/1 -> Sweep Logic/2(sweep)
  [exit_id] -> Sweep Logic/1(exit_id)
  Nav Leg/6(exit_id) -> [exit_id]
  [entry_id] -> Proximity Distance/5(entry_id)
  Nav Leg/5(entry_id) -> [entry_id]
  Mission Director/4(state_flg) -> [state_flg]
  [sweep_flg] -> Mission Director/8(sweep_flg)
  [entry_id] -> Mission Director/6(fly_over_flg)
  [fly_away_flg] -> Mission Director/7(fly_away_flg)
  [orbit_flg] -> Mission Director/5(orbit_flg)
  [orbit_len] -> Mission Director/4(orbit_time)
  [d2n] -> Mission Director/2(d2n)
  [leg_state] -> leg_state/1
  Nav Leg/1(leg_state) -> [leg_state]
  [turn_rad] -> Fly Away Detection/3(turn_rad)
  Proximity Distance/4(turn_rad) -> [turn_rad]
  Detect Increase/1 -> Fly Away Detection/2(retreating)
  [d2n] -> Fly Away Detection/1(d2n), Detect Increase/1
  [prox_dist] -> Mux/1
  Mux/1 -> Scope1/3
  [d2n] -> Mux/2
  d2n/1 -> [d2n]
  [leg_state] -> Proximity Distance/4(leg_state)
  [nav_mode] -> Nav Leg/3(nav_mode)
  [av_state] -> Nav Leg/1(av_state)
  [av_state] -> Proximity Distance/2(av_state)
  av_state/1 -> [av_state]
  wind_state/1 -> Proximity Distance/3(wnd_state)
  [prox_dist] -> Mission Director/3(prox_dist)
  Proximity Distance/1(prox_dist) -> [prox_dist]
  Proximity Distance/3(orbit_len) -> [orbit_len]
  Proximity Distance/2(orbit_flg) -> [orbit_flg]
  [orbit_state] -> Proximity Distance/1(orbit_state)
  [orbit_state] -> orbit_state/1
  [state_flg] -> Scope1/2  "State Flag"
  [nav_mode] -> Scope1/1  "Nav Mode"
  [msn_rst] -> Memory2/1
  [nav_mode] -> nav_mode/1
  Mission Director/3(msn_rst) -> [msn_rst]
  Mission Director/2(nav_mode) -> [nav_mode]
  Constant2/1 -> Mission Director/1(Ovrd)
  MATLAB Function/1(wp_to) -> Nav Leg/2(wp_to)  "To WP"
  Memory3/1 -> MATLAB Function/2(wp_upd_old)
  Mission Director/1(wp_upd) -> MATLAB Function/1(wp_upd), Memory3/1
  Constant3/1 -> MATLAB Function/3(wp_entry)
  [curr_wp] -> MATLAB Function/4(wp_curr)
  [next_wp] -> MATLAB Function/5(wp_next)
  Nav Leg/3(next_wp) -> [next_wp]
  Nav Leg/2(curr_wp) -> [curr_wp]
  Nav Leg/4(orbit_state) -> [orbit_state]

== system hapsrav_library/Cmd - Parametric/Chi Cmd/Subsystem/Azimuth angle not bounded by 0, 2pi ==
  sun_az_rad : Inport
  Compare To Constant : simulink/Logic and Bit Operations/Compare To Constant  relop=<=  const=-1.9*pi  OutDataTypeStr=boolean
  Compare To Constant1 : simulink/Logic and Bit Operations/Compare To Constant  relop=>=  const=1.9*pi  OutDataTypeStr=boolean
  Counter : Subsystem
  Counter1 : Subsystem
  Delay{1..4} (4 alike) : Delay  DelayLength=1  InitialCondition=0
  Gain1 : Gain  Gain=2*pi
  Sum1 : Sum  Inputs=|+-
  Sum2 : Sum  Inputs=|+-
  Sum3 : Sum  Inputs=|++
  2*pi*i : Outport
  wires:
  Sum3/1 -> Gain1/1
  Delay2/1 -> Sum1/2
  sun_az_rad/1 -> Sum2/1, Delay1/1, Sum1/1, Delay2/1
  Delay3/1 -> Counter1/1(i)
  Sum1/1 -> Compare To Constant1/1
  Compare To Constant1/1 -> Counter1/Trigger
  Counter1/1(i-1) -> Sum3/2, Delay3/1
  Gain1/1 -> 2*pi*i/1
  Delay4/1 -> Counter/1(i)
  Delay1/1 -> Sum2/2
  Sum2/1 -> Compare To Constant/1
  Counter/1(i+1) -> Sum3/1, Delay4/1
  Compare To Constant/1 -> Counter/Trigger

== system hapsrav_library/Cmd - Parametric/Chi Cmd/Subsystem/Circular Orbit ==
  chi_cmd_in : Inport
  t : Inport  Port=2
  Enable : EnablePort  StatesWhenEnabling=reset  ShowOutputPort=on
  Constant : Constant  Value=vtas_init
  Constant1 : Constant  Value=pi/(turn_time_circle)
  Constant2 : Constant  Value=Wdir
  Discrete-Time Integrator : DiscreteIntegrator  IntegratorMethod=Integration: Trapezoidal  ExternalReset=rising  InitialConditionSetting=State (most efficient)  SampleTime=dT  ICPrevOutput=DiscIntNeverNeededParam  ICPrevScaledInput=DiscIntNeverNeededParam
  Divide : Product  Inputs=*/
  Divide1 : Product  Inputs=**
  Gain : Gain  Gain=Wmag
  ICs for turn : Subsystem  TreatAsAtomicUnit=on
  Sum1 : Sum  Inputs=|++
  Sum2 : Sum  Inputs=|++
  Sum3 : Sum  Inputs=+-|
  To Workspace : ToWorkspace  VariableName=chi_rate_circular_cmd  SampleTime=-1
  Trigonometric Function : Trigonometry  Operator=cos
  chi_cmd : Outport
  wires:
  Divide/1 -> Divide1/1
  Divide1/1 -> Discrete-Time Integrator/1, To Workspace/1
  Constant2/1 -> Sum3/1
  Trigonometric Function/1 -> Gain/1
  Sum3/1 -> Trigonometric Function/1
  Gain/1 -> Sum1/1
  Sum1/1 -> Divide/1
  Constant1/1 -> Divide1/2
  ICs for turn/1(t0) -> Discrete-Time Integrator/2
  Discrete-Time Integrator/1 -> Sum2/1
  Constant/1 -> Divide/2, Sum1/2
  Enable/1 -> ICs for turn/Trigger
  ICs for turn/2(chi0) -> Sum2/2
  chi_cmd_in/1 -> Sum3/2, ICs for turn/2(chi_cmd)
  t/1 -> ICs for turn/1(t)
  Sum2/1 -> chi_cmd/1

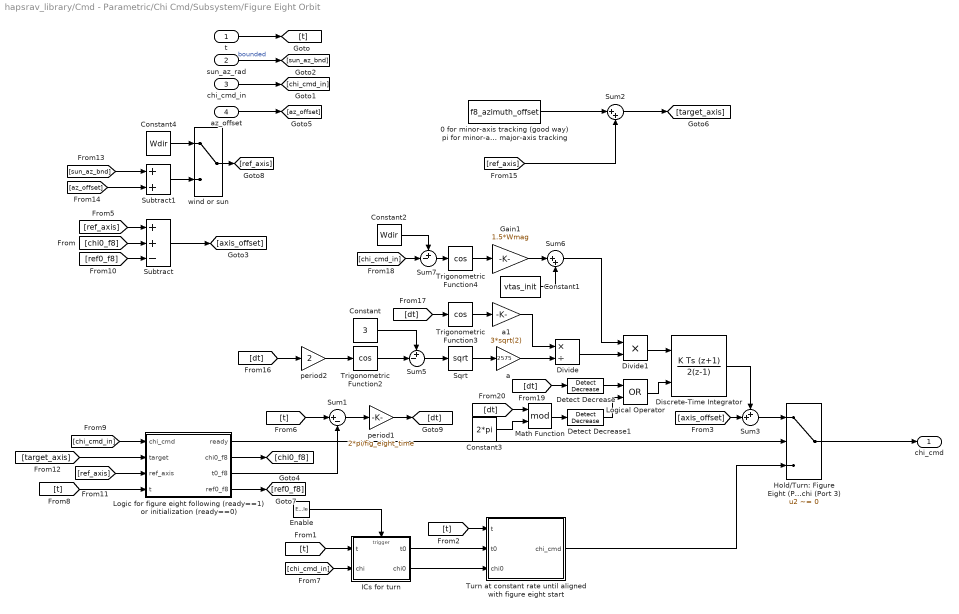
== system hapsrav_library/Cmd - Parametric/Chi Cmd/Subsystem/Figure Eight Orbit ==
  t : Inport
  sun_az_rad : Inport  Port=2
  chi_cmd_in : Inport  Port=3
  az_offset : Inport  Port=4
  Enable : EnablePort  StatesWhenEnabling=reset  ShowOutputPort=on
  0 for minor-axis tracking (good way) pi for minor-axis tracking (bad way) pi/2 for major-axis tracking : Constant  Value=f8_azimuth_offset
  Constant : Constant  Value=3
  Constant1 : Constant  Value=vtas_init
  Constant2 : Constant  Value=Wdir
  Constant3 : Constant  Value=2*pi
  Constant4 : Constant  Value=Wdir
  Detect Decrease : simulink/Logic and Bit Operations/Detect Decrease  vinit=0.0  OutDataTypeStr=boolean
  Detect Decrease1 : simulink/Logic and Bit Operations/Detect Decrease  vinit=0.0  OutDataTypeStr=boolean
  Discrete-Time Integrator : DiscreteIntegrator  IntegratorMethod=Integration: Trapezoidal  ExternalReset=rising  InitialConditionSetting=State (most efficient)  SampleTime=dT  ICPrevOutput=DiscIntNeverNeededParam  ICPrevScaledInput=DiscIntNeverNeededParam
  Divide : Product  Inputs=*/
  Divide1 : Product  Inputs=**
  Gain1 : Gain  Gain=1.5*Wmag
  Hold/Turn: Figure Eight (Port 1) Initialization: constant d1chi (Port 3) : Switch  Criteria=u2 ~= 0
  ICs for turn : Subsystem  TreatAsAtomicUnit=on
  Logic for figure eight following (ready==1) or initialization (ready==0) : Subsystem
  Logical Operator : Logic  Operator=OR  AllPortsSameDT=off  OutDataTypeStr=boolean
  Math Function : Math  Operator=mod  SaturateOnIntegerOverflow=on
  Sqrt : Sqrt  SaturateOnIntegerOverflow=on
  Subtract : Sum  Inputs=++-
  Subtract1 : Sum
  Sum1 : Sum  Inputs=|+-
  Sum2 : Sum  Inputs=|++
  Sum3 : Sum  Inputs=++|
  Sum5 : Sum  Inputs=+-|
  Sum6 : Sum  Inputs=|++
  Sum7 : Sum  Inputs=+-|
  Trigonometric Function2 : Trigonometry  Operator=cos
  Trigonometric Function3 : Trigonometry  Operator=cos
  Trigonometric Function4 : Trigonometry  Operator=cos
  Turn at constant rate until aligned with figure eight start : Subsystem
  a : Gain  Gain=2575
  a1 : Gain  Gain=3*sqrt(2)
  period1 : Gain  Gain=2*pi/fig_eight_time
  period2 : Gain  Gain=2
  wind or sun : ManualSwitch
  chi_cmd : Outport
  wires:
  Subtract1/1 -> wind or sun/2
  Constant4/1 -> wind or sun/1
  Gain1/1 -> Sum6/1
  Constant3/1 -> Math Function/2
  [dt] -> Math Function/1
  Detect Decrease1/1 -> Logical Operator/2
  Math Function/1 -> Detect Decrease1/1
  [dt] -> Detect Decrease/1
  Detect Decrease/1 -> Logical Operator/1
  Logical Operator/1 -> Discrete-Time Integrator/2
  Sum6/1 -> Divide1/1
  Trigonometric Function4/1 -> Gain1/1
  Constant1/1 -> Sum6/2
  [chi_cmd_in] -> Sum7/2
  Sum7/1 -> Trigonometric Function4/1
  Constant2/1 -> Sum7/1
  Divide/1 -> Divide1/2
  Discrete-Time Integrator/1 -> Sum3/1
  a/1 -> Divide/2
  Trigonometric Function3/1 -> a1/1
  Trigonometric Function2/1 -> Sum5/2
  [dt] -> Trigonometric Function3/1
  a1/1 -> Divide/1
  Sum5/1 -> Sqrt/1
  Constant/1 -> Sum5/1
  period2/1 -> Trigonometric Function2/1
  [dt] -> period2/1
  period1/1 -> [dt]
  Sqrt/1 -> a/1
  Divide1/1 -> Discrete-Time Integrator/1
  [axis_offset] -> Sum3/2
  Sum3/1 -> Hold/Turn: Figure Eight (Port 1) Initialization: constant d1chi (Port 3)/1
  Logic for figure eight following (ready==1) or initialization (ready==0)/3(t0_f8) -> Sum1/2
  [t] -> Sum1/1
  Sum1/1 -> period1/1
  wind or sun/1 -> [ref_axis]
  [az_offset] -> Subtract1/2
  [sun_az_bnd] -> Subtract1/1
  [ref0_f8] -> Subtract/3
  [chi0_f8] -> Subtract/2
  [ref_axis] -> Subtract/1
  Subtract/1 -> [axis_offset]
  Logic for figure eight following (ready==1) or initialization (ready==0)/4(ref0_f8) -> [ref0_f8]
  Hold/Turn: Figure Eight (Port 1) Initialization: constant d1chi (Port 3)/1 -> chi_cmd/1
  [t] -> Logic for figure eight following (ready==1) or initialization (ready==0)/4(t)
  Sum2/1 -> [target_axis]
  [ref_axis] -> Sum2/2
  [target_axis] -> Logic for figure eight following (ready==1) or initialization (ready==0)/2(target)
  [chi_cmd_in] -> Logic for figure eight following (ready==1) or initialization (ready==0)/1(chi_cmd)
  Logic for figure eight following (ready==1) or initialization (ready==0)/1(ready) -> Hold/Turn: Figure Eight (Port 1) Initialization: constant d1chi (Port 3)/2
  Enable/1 -> ICs for turn/Trigger
  [ref_axis] -> Logic for figure eight following (ready==1) or initialization (ready==0)/3(ref_axis)
  az_offset/1 -> [az_offset]
  Logic for figure eight following (ready==1) or initialization (ready==0)/2(chi0_f8) -> [chi0_f8]
  [t] -> Turn at constant rate until aligned with figure eight start/1(t)
  ICs for turn/2(chi0) -> Turn at constant rate until aligned with figure eight start/3(chi0)
  [t] -> ICs for turn/1(t)
  [chi_cmd_in] -> ICs for turn/2(chi)
  ICs for turn/1(t0) -> Turn at constant rate until aligned with figure eight start/2(t0)
  Turn at constant rate until aligned with figure eight start/1(chi_cmd) -> Hold/Turn: Figure Eight (Port 1) Initialization: constant d1chi (Port 3)/3
  chi_cmd_in/1 -> [chi_cmd_in]
  0 for minor-axis tracking (good way) pi for minor-axis tracking (bad way) pi/2 for major-axis tracking/1 -> Sum2/1
  sun_az_rad/1 -> [sun_az_bnd]  "bounded"
  t/1 -> [t]

== system hapsrav_library/Cmd - Parametric/Chi Cmd/Subsystem/Racetrack Orbit ==
  t : Inport
  chi_cmd_in : Inport  Port=2
  sun_az_rad : Inport  Port=3
  Enable : EnablePort  StatesWhenEnabling=reset
  Delay1 : Delay  DelayLength=1  InitialCondition=chi_init-pi/2
  Hold/Turn: Constant chi (Port 1) Constant d1chi (Port 3) : Switch  Criteria=u2 ~= 0
  ICs for turn : Subsystem  TreatAsAtomicUnit=on
  Periodic Climb/Glide : Subsystem
  Pulsing Logic: 1 for hold course 0 for turn : Subsystem
  Turn at constant rate : Subsystem
  chi_cmd : Outport
  up_or_down : Outport  Port=2
  wires:
  Periodic Climb/Glide/1(up_or_down) -> up_or_down/1
  [sun_az_rad] -> Periodic Climb/Glide/2(sun_az_rad)
  [chi_cmd_in] -> Periodic Climb/Glide/1(chi_cmd_in)
  Pulsing Logic: 1 for hold course 0 for turn/1(hold (bool)) -> Hold/Turn: Constant chi (Port 1) Constant d1chi (Port 3)/2, Periodic Climb/Glide/3(hold), ICs for turn/Trigger
  ICs for turn/1(t0) -> Turn at constant rate/2(t0)
  ICs for turn/2(chi0) -> Turn at constant rate/3(chi0), Delay1/1
  [chi_cmd_in] -> Hold/Turn: Constant chi (Port 1) Constant d1chi (Port 3)/1
  t/1 -> [t]
  chi_cmd_in/1 -> [chi_cmd_in]
  [t] -> Turn at constant rate/1(t)
  [chi_cmd_in] -> Pulsing Logic: 1 for hold course 0 for turn/2(chi)
  Delay1/1 -> Pulsing Logic: 1 for hold course 0 for turn/4(last_chi)
  [chi_cmd_in] -> ICs for turn/2(chi)
  [t] -> ICs for turn/1(t)
  Hold/Turn: Constant chi (Port 1) Constant d1chi (Port 3)/1 -> chi_cmd/1
  [t] -> Pulsing Logic: 1 for hold course 0 for turn/1(t)
  Turn at constant rate/1(chi_cmd) -> Hold/Turn: Constant chi (Port 1) Constant d1chi (Port 3)/3
  [sun_az_rad] -> Pulsing Logic: 1 for hold course 0 for turn/3(sun_az_rad)
  sun_az_rad/1 -> [sun_az_rad]

== system hapsrav_library/hapsrav_main/Kinematic 6DOF/Aero/CL vs AoA ==
  Vtas : Inport
  gamma : Inport  Port=2
  qS : Inport  Port=3
  alt : Inport  Port=4
  phi : Inport  Port=5
  CD LUT : Subsystem
  Constant : Constant  Value=earth_rho
  Divide : Product  Inputs=*/
  Divide1 : Product  Inputs=*/
  Divide2 : Product  Inputs=*/
  Gain1 : Gain  Gain=M*g
  Gain2 : Gain  Gain=M
  Math Function2 : Math  Operator=square  SaturateOnIntegerOverflow=on
  Sum : Sum
  Sum1 : Sum  Inputs=|++
  Sum2 : Sum  Inputs=|++
  Trigonometric Function : Trigonometry  Operator=cos
  Trigonometric Function1 : Trigonometry  Operator=cos
  alpha RLUT : Subsystem
  CL : Outport
  CD : Outport  Port=2
  alpha : Outport  Port=3
  theta : Outport  Port=4
  wires:
  Math Function2/1 -> Gain2/1
  Divide/1 -> Sum1/1
  Constant/1 -> Sum/1
  Vtas/1 -> Math Function2/1
  Sum1/1 -> Divide2/1
  Gain1/1 -> Sum1/2
  Trigonometric Function/1 -> Gain1/1
  Sum/1 -> Divide/2
  Gain2/1 -> Divide/1
  qS/1 -> Divide2/2
  [alpha] -> Sum2/2
  Sum2/1 -> theta/1
  Divide2/1 -> Divide1/1
  phi/1 -> Trigonometric Function1/1
  Trigonometric Function1/1 -> Divide1/2
  Divide1/1 -> [CL]
  [alpha] -> alpha/1
  gamma/1 -> [gamma]
  [gamma] -> Trigonometric Function/1
  [gamma] -> Sum2/1
  alpha RLUT/1(alpha_rad) -> CD LUT/1(alpha), [alpha]
  [CL] -> alpha RLUT/2(CL)
  alt/1 -> [alt]
  [alt] -> alpha RLUT/1(alt)
  [alt] -> Sum/2
  [CD] -> CD/1
  CD LUT/1(CD) -> [CD]
  [alt] -> CD LUT/2(alt)
  [CL] -> CL/1
